simulink model "mpc_model_classical"  (R2019a)
settings: Solver=VariableStepAuto  StartTime=0.0  StopTime=Tfinal  RelTol=1e-3
values from neighbouring files (symbols this model uses):
  A = [-0.0285 -0.0014; -0.0371 -0.1476]    [model.m]
  DCLINK_Cap = 1000e-12    (= 1e-09)    [mpc_model_parameters.m]    (also in mpc_model_parameters_dual_module.m = 0.001)
  FaultTime = 50    [mpc_model_parameters.m]
  FluxPM = MeanInducedVoltagePeak/(2*pi*100)    [mpc_model_parameters.m]    (also in mpc_model_parameters_dual_module.m)
  Inertia = 1e-2    (= 0.01)    [mpc_model_parameters.m]    (also in mpc_model_parameters_dual_module.m)
  intangle1 = 0    [mpc_model_parameters.m]    (also in mpc_model_parameters_dual_module.m)
  Ki = 8    [mpc_model_parameters_dual_module.m]
  Kp = 0.8    [mpc_model_parameters_dual_module.m]
  ma = 0.9    [mpc_model_parameters.m]    (also in mpc_model_parameters_dual_module.m)
  MeanLd = (1/12)*(Module1Phase_A_Ld+Module1Phase_B_Ld+Module1Phase_C_Ld+     Module2Phase_A_Ld+Module2Phase_B_Ld+Module2Phase_C_Ld+     Module3Phase_A_Ld+Module3Phase_B_Ld+Module3Phase_C_Ld+     Module4Phase_A_Ld+Module4Phase_B_Ld+Module4Phase_C_Ld)    [mpc_model_parameters.m]    (also in mpc_model_parameters_dual_module.m)
  MeanLq = (1/12)*(Module1Phase_A_Lq+Module1Phase_B_Lq+Module1Phase_C_Lq+     Module2Phase_A_Lq+Module2Phase_B_Lq+Module2Phase_C_Lq+     Module3Phase_A_Lq+Module3Phase_B_Lq+Module3Phase_C_Lq+     Module4Phase_A_Lq+Module4Phase_B_Lq+Module4Phase_C_Lq)    [mpc_model_parameters.m]    (also in mpc_model_parameters_dual_module.m)
  PI_Frequency = 5000    [mpc_model_parameters_dual_module.m]
  PI_Sat = iqrated*2    [mpc_model_parameters_dual_module.m]
  PI_Ts = 1/PI_Frequency    (= 0.0002)    [mpc_model_parameters_dual_module.m]
  PolePairs = 10    [mpc_model_parameters.m]    (also in mpc_model_parameters_dual_module.m)
  ref_frequency = 100*pi    (= 314.159265359)    [mpc_model_parameters.m]    (also in mpc_model_parameters_dual_module.m)
  Rin = 1e-3    (= 0.001)    [mpc_model_parameters.m]    (also in mpc_model_parameters_dual_module.m)
  Rs = 0.531    [Loss_Distribution.m]    (also in MPC_id_iq.m; mpc_model_parameters.m = 0.321; mpc_model_parameters_dual_module.m = 0.539)
  Sampling_time = 1e-6    (= 1e-06)    [mpc_model_parameters.m]    (also in mpc_model_parameters_dual_module.m)
  SpeedRef1 = 50    [mpc_model_parameters.m]    (also in mpc_model_parameters_dual_module.m = 35)
  SpeedRef2 = 100    [mpc_model_parameters.m]    (also in mpc_model_parameters_dual_module.m = 35)
  SpeedRefUpdateTime = 0.25    [mpc_model_parameters.m]    (also in mpc_model_parameters_dual_module.m = 1.75)
  Tload1 = 5    [mpc_model_parameters.m]    (also in mpc_model_parameters_dual_module.m = 30)
  Tload2 = 10    [mpc_model_parameters.m]    (also in mpc_model_parameters_dual_module.m = 63.6619772368)
  TloadUpdateTime = 0.5    [mpc_model_parameters.m]    (also in mpc_model_parameters_dual_module.m)
  Vdc = 50    [mpc_model_parameters.m]    (also in mpc_model_parameters_dual_module.m = 40)
  Vin = Vdc + Rin*(Pout/Vdc)    (= 50.04)    [mpc_model_parameters.m]    (also in mpc_model_parameters_dual_module.m = 40.05)
  ViscousFriction = 1e-3    (= 0.001)    [mpc_model_parameters.m]    (also in mpc_model_parameters_dual_module.m)
undefined symbols (not defined in the file or in its folder): DiscIntNeverNeededParam
libraries: powerlib x16, dspswit3 x8, powerlib_meascontrol x5, simulink x1, dspsigops x1
settings Model: Creator=hakan  LastModifiedBy=hakan
settings SolverCC: ZeroCrossAlgorithm=Adaptive
settings DebuggingCC: IgnoredZcDiagnostic=none

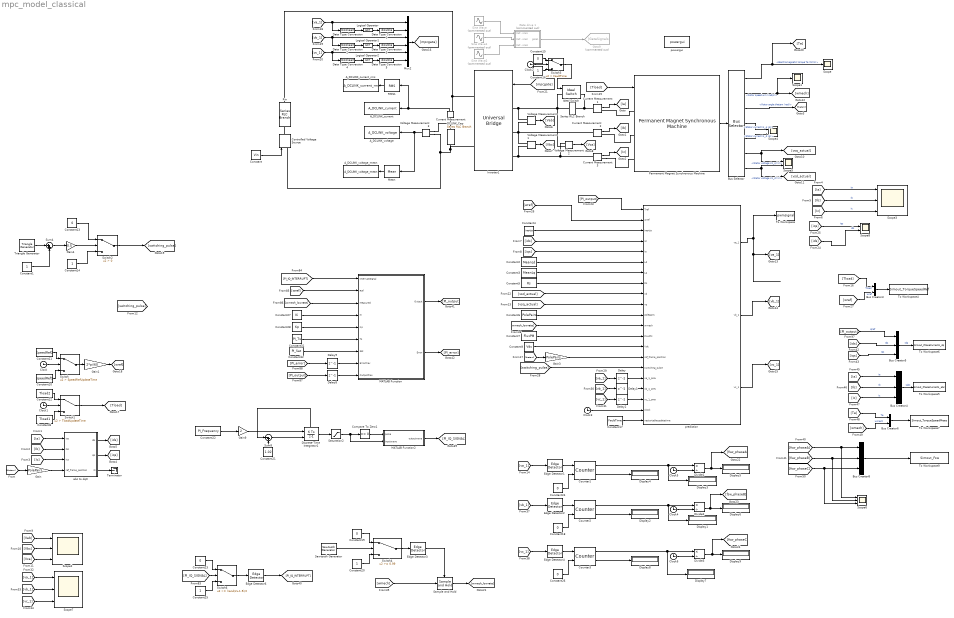
== system mpc_model_classical ==
  A_DCLINK_current : ToWorkspace  VariableName=A_DCLINK_current  SaveFormat=Structure With Time  SampleTime=-1
  A_DCLINK_current_rms : ToWorkspace  VariableName=A_DCLINK_current_rms  SaveFormat=Structure With Time  SampleTime=-1
  A_DCLINK_voltage : ToWorkspace  VariableName=A_DCLINK_voltage  SaveFormat=Structure With Time  SampleTime=-1
  A_DCLINK_voltage_mean : ToWorkspace  VariableName=A_DCLINK_voltage_mean  SaveFormat=Structure With Time  SampleTime=-1
  Bus Creator3 : BusCreator  Inputs=2
  Bus Creator4 : BusCreator  Inputs=3
  Bus Creator5 : BusCreator  Inputs=3
  Bus Creator6 : BusCreator  Inputs=2
  Bus Creator8 : BusCreator  Inputs=3
  Bus Selector : BusSelector  OutputSignals=Electromagnetic torque Te (N*m),Rotor speed wm (rad/s),Rotor angle thetam (rad),Stator current is_q (A),Stator current is_d (A),Stator voltage Vs_q (V),Stator voltage Vs_d (V)
  Clock{,1..6} (7 alike) : Clock
  Compare To Zero1 : simulink/Logic and Bit Operations/Compare To Zero  relop===  OutDataTypeStr=boolean
  Constant : Constant  Value=Vin
  Constant{1,14,16,20,25} (5 alike) : Constant
  Constant10 : Constant  Value=SpeedRef1
  Constant11 : Constant  Value=SpeedRef2
  Constant12 : Constant  Value=Tload2
  Constant{13,15,18..19,23..24,26} (7 alike) : Constant  Value=0
  Constant17 : Constant  Value=FaultTime
  Constant2 : Constant  Value=MeanLd
  Constant21 : Constant  Value=1.02
  Constant22 : Constant  Value=PI_Frequency
  Constant27 : Constant  Value=Ki
  Constant28 : Constant  Value=Kp
  Constant3 : Constant  Value=MeanLq
  Constant31 : Constant  Value=PI_Ts
  Constant32 : Constant  Value=PI_Sat
  Constant4 : Constant  Value=Inertia
  Constant5 : Constant  Value=Rs
  Constant6 : Constant  Value=PolePairs
  Constant7 : Constant  Value=FluxPM
  Constant8 : Constant  Value=Tload1
  Constant9 : Constant  Value=Vdc
  Controlled Voltage Source : powerlib/Electrical Sources/Controlled Voltage Source  Initialize=on  Source_Type=DC  Amplitude=0  Phase=0  Frequency=0  Measurements=None
      settings: SourceProductName=Simscape Electrical
  Counter1 : dspswit3/Counter  Direction=Up  CountEvent=Rising edge  CounterSize=User defined  MaxCount=9999999999999999999  InitialCount=0  Output=Count and Hit  HitValue=32  ResetInput=on  SamplesPerFrame=1  Ts=1  CntDtype=double  HitDtype=Logical
  Counter2 : dspswit3/Counter  Direction=Up  CountEvent=Rising edge  CounterSize=User defined  MaxCount=9999999999999999999  InitialCount=0  Output=Count and Hit  HitValue=32  ResetInput=on  SamplesPerFrame=1  Ts=1  CntDtype=double  HitDtype=Logical
  Counter3 : dspswit3/Counter  Direction=Up  CountEvent=Rising edge  CounterSize=User defined  MaxCount=9999999999999999999  InitialCount=0  Output=Count and Hit  HitValue=32  ResetInput=on  SamplesPerFrame=1  Ts=1  CntDtype=double  HitDtype=Logical
  Current Measurement{,1..3} (4 alike) : powerlib/Measurements/Current Measurement  PhasorSimulation=off  OutputType=Complex  PSBequivalent=0
      settings: SourceProductName=Simscape Electrical
  DCLINK_Cap : powerlib/Elements/Series RLC Branch  LConnTagsString=__new0  RConnTagsString=__new0  BranchType=C  Resistance=1  Inductance=1e-3  SetiL0=off  InitialCurrent=0  Capacitance=DCLINK_Cap  Setx0=on  InitialVoltage=Vin  Measurements=None
      settings: SourceProductName=Simscape Electrical
  Data Type Conversion : DataTypeConversion  OutDataTypeStr=boolean
  Data Type Conversion1 : DataTypeConversion  OutDataTypeStr=double
  Data Type Conversion2 : DataTypeConversion  OutDataTypeStr=boolean
  Data Type Conversion3 : DataTypeConversion  OutDataTypeStr=double
  Data Type Conversion4 : DataTypeConversion  OutDataTypeStr=boolean
  Data Type Conversion5 : DataTypeConversion  OutDataTypeStr=double
  Delay{,1..2,8..9} (5 alike) : Delay  DelayLength=1
  Discrete-Time Integrator1 : DiscreteIntegrator  ExternalReset=falling  SampleTime=Sampling_time  UpperSaturationLimit=1  LowerSaturationLimit=0  ShowStatePort=on  ICPrevOutput=DiscIntNeverNeededParam  ICPrevScaledInput=DiscIntNeverNeededParam
  Display{1..9} (9 alike) : Display
  Divide1 : Product  Inputs=*/
  Divide2 : Product  Inputs=*/
  Divide3 : Product  Inputs=*/
  Edge Detector{1..4,6} (5 alike) : dspswit3/Edge Detector  InputProcessing=Columns as channels (frame based)
      settings: SourceProductName=DSP System Toolbox  SourceProductBaseCode=DS
  Gain : Gain  Gain=PolePairs
  Gain1 : Gain  Gain=2*pi/60
  Gain3 : Gain  Gain=PolePairs
  Gain4 : Gain  Gain=0.5
  Gain9 : Gain  Gain=2
  Gate drive 1 : Subsystem  Commented=on
  Goto9 : Goto  Commented=on  GotoTag=GateSignals
  Ideal Switch : powerlib/Power Electronics/Ideal Switch  Ron=0.001  Lon=0  IC=0  Rs=1e5  Cs=inf  Measurements=on
      settings: SourceProductName=Simscape Electrical
  Inverter1 : powerlib/Power Electronics/Universal Bridge  Arms=3  SnubberResistance=1e5  SnubberCapacitance=inf  Device=IGBT / Diodes  Ron=0.65e-3  Lon=0  ForwardVoltages="[  0  0  ]"  ForwardVoltage=0  GTOparameters=[ 10e-6 , 20e-6 ]  IGBTparameters=[ 1e-6 , 2e-6 ]  Measurements=All voltages and currents  Measurements_2=None  converterType=Rectifier
      settings: SourceProductName=Simscape Electrical
  Logical Operator : Logic  Operator=NOT  AllPortsSameDT=off  OutDataTypeStr=boolean
  Logical Operator1 : Logic  Operator=NOT  AllPortsSameDT=off  OutDataTypeStr=boolean
  Logical Operator2 : Logic  Operator=NOT  AllPortsSameDT=off  OutDataTypeStr=boolean
  MATLAB Function : MATLAB Function  TreatAsAtomicUnit=on
  MATLAB Function2 : MATLAB Function  TreatAsAtomicUnit=on
  Mean : powerlib_meascontrol/Measurements/Mean  Freq=THD_mean_frequency  Vinit=0  Ts=0
      settings: SourceProductName=Simscape Electrical
  Mux2 : Mux  Inputs=6
  Permanent Magnet Synchronous Machine : powerlib/Machines/Permanent Magnet Synchronous Machine  NbPhases=3  FluxDistribution=Sinusoidal  RotorType=Round  MechanicalLoad=Torque Tm  PresetModel=No  ShowDetailedParameters=on  MeasurementBus=off  Resistance=Rs  Inductance=8.5e-3  dqInductances=[3.1e-3,3.6e-3]  La=Ls  MachineConstant=Voltage Constant (V_peak L-L / krpm)  Flux=0.18074  VoltageCst=VoltageConstant  TorqueCst=2.7111  Flat=120  Mechanical=[Inertia ViscousFriction PolePairs 0]  PolePairs=4  InitialConditions=[0,0, 0,0]  InitialConditions5ph=[0 0 0 0 0 0]  TsPowergui=0  TsBlock=-1  RefAngle=90 degrees behind phase A axis (modified Park)
  RMS1 : powerlib_meascontrol/Measurements/RMS  TrueRMS=on  Freq=Load_Nominal_Freq  RMSInit=10  Ts=0
      settings: SourceProductName=Simscape Electrical
  Rin : powerlib/Elements/Series RLC Branch  LConnTagsString=__new0  RConnTagsString=__new0  BranchType=R  Resistance=Rin  Inductance=1e-3  SetiL0=off  InitialCurrent=0  Capacitance=1000e-6  Setx0=off  InitialVoltage=0  Measurements=None
      settings: SourceProductName=Simscape Electrical
  Sample and Hold : dspsigops/Sample and Hold  trig=Rising edge  initCond=0  latchinput=off
  Saturation2 : Saturate  UpperLimit=1  LowerLimit=0
  Sawtooth Generator : powerlib_meascontrol/Pulse & Signal Generators/Sawtooth Generator  Freq=1000  Phase=180  Ts=0
      settings: SourceProductName=Simscape Electrical
  Scope : Scope
  Scope1 : Scope
  Scope{2..3,6..7} (4 alike) : Scope  NumInputPorts=3
  Scope4 : Scope  NumInputPorts=2
  Scope5 : Scope  NumInputPorts=2
  Scope8 : Scope  NumInputPorts=2
  Series RLC Branch : powerlib/Elements/Series RLC Branch  LConnTagsString=__new0  RConnTagsString=__new0  BranchType=R  Resistance=5000  Inductance=1e-3  SetiL0=off  InitialCurrent=0  Capacitance=1e-6  Setx0=off  InitialVoltage=0  Measurements=None
      settings: SourceProductName=Simscape Electrical
  Sine Wave : Sin  Commented=on  Amplitude=ma  Frequency=ref_frequency  SampleTime=0
  Sine Wave1 : Sin  Commented=on  Amplitude=ma  Frequency=ref_frequency  Phase=-2*pi/3  SampleTime=0
  Sine Wave2 : Sin  Commented=on  Amplitude=ma  Frequency=ref_frequency  Phase=2*pi/3  SampleTime=0
  Sum4 : Sum  Inputs=|++
  Sum8 : Sum  Inputs=|-+
  Switch : Switch  Criteria=u2 > Threshold  Threshold=SpeedRefUpdateTime
  Switch1 : Switch  Criteria=u2 > Threshold  Threshold=TloadUpdateTime
  Switch2 : Switch  Criteria=u2 > Threshold
  Switch3 : Switch  Criteria=u2 > Threshold  Threshold=FaultTime
  Switch4 : Switch  Threshold=0.99
  Switch6 : Switch  Threshold=(rand/2+1.5)/2
  Terminator : Terminator
  To Workspace : ToWorkspace  VariableName=pwmsignal  SaveFormat=Timeseries  SampleTime=-1
  To Workspace4 : ToWorkspace  VariableName=Simout_TorqueSpeedRef  SaveFormat=Timeseries  SampleTime=-1
  To Workspace5 : ToWorkspace  VariableName=Simout_PhaseCurrents_abc  SaveFormat=Timeseries  SampleTime=-1
  To Workspace6 : ToWorkspace  VariableName=Simout_PhaseCurrents_dq  SaveFormat=Timeseries  SampleTime=-1
  To Workspace7 : ToWorkspace  VariableName=Simout_TorqueSpeedMeas  SaveFormat=Timeseries  SampleTime=-1
  To Workspace9 : ToWorkspace  VariableName=Simout_Fsw  SaveFormat=Timeseries  SampleTime=-1
  Triangle Generator : powerlib_meascontrol/Pulse & Signal Generators/Triangle Generator  Freq=sw_frequency  Phase=0  Ts=Sampling_time
      settings: SourceProductName=Simscape Electrical
  Voltage Measurement{,1..3} (4 alike) : powerlib/Measurements/Voltage Measurement  PhasorSimulation=off  OutputType=Complex  PSBequivalent=0
      settings: SourceProductName=Simscape Electrical
  abc to dq0 : MATLAB Function  TreatAsAtomicUnit=on
  powergui : powerlib/powergui  Priority=1  SimulationMode=Discrete  SampleTime=Sampling_time  frequency=60  Iterations=50  frequencyindice=0  Pbase=100e6  ErrMax=1e-4  UnitsV=kV  UnitsW=MW  buscounter=0  FunctionMessages=off  echomessages=off  EnableUseOfTLC=off  CurrentSourceSwitches=off  DisableSnubberDevices=off  DisableRonSwitches=off  DisableVfSwitches=off  DisplayEquations=off  AutomaticDiscreteSolvers=off  SolverType=Tustin/Backward Euler (TBE)  Interpol=off  ExternalGateDelay=off  methode=off  Ts=100  x0status=blocks  SPID=on  SwTol=0  HookPort=off  NonlinearTolerance=0  nMaxIteration=15  ContinueOnMaxIteration=off  RestoreLinks=warning  ResistiveCurrentMeasurement=off  Frange=[0:2:500]  Ylog=off  Xlog=on  ShowGrid=off  save=off  variable=ZData  structure=0  ZoomFFT=off  StartTime=0.0  cycles=1  DisplayStyle=1  fundamental=60  FreqAxis=off  MaxFrequency=1000  frequencyindicesteady=1  RmsSteady=1  display=off
      settings: SourceProductName=Simscape Electrical
  prediction : MATLAB Function  TreatAsAtomicUnit=on
  wires:
  Voltage Measurement3/1 -> Mean/1, A_DCLINK_voltage/1
  RMS1/1 -> A_DCLINK_current_rms/1
  Constant/1 -> Controlled Voltage Source/1
  Mean/1 -> A_DCLINK_voltage_mean/1
  Current Measurement/1 -> RMS1/1, A_DCLINK_current/1
  Gate drive 1/1(gate1) -> Goto9/1
  Permanent Magnet Synchronous Machine/1 -> Bus Selector/1
  Bus Selector/1 -> [Te], Scope/1  "<Electromagnetic torque Te (N*m)>"
  Bus Selector/2 -> [wmech], Scope1/1  "<Rotor speed wm (rad/s)>"
  Sine Wave1/1 -> Gate drive 1/2(Reference2)
  Sine Wave/1 -> Gate drive 1/1(Reference1)
  Sine Wave2/1 -> Gate drive 1/3(Reference3)
  Current Measurement1/1 -> [Ia]
  Current Measurement2/1 -> [Ib]
  Current Measurement3/1 -> [Ic]
  Bus Selector/3 -> [thetam]  "<Rotor angle thetam (rad)>"
  [thetam] -> Gain/1
  [Ia] -> abc to dq0/1(ias)
  [Ib] -> abc to dq0/2(ibs)
  [Ic] -> abc to dq0/3(ics)
  Gain/1 -> abc to dq0/4(ref_frame_position)
  [Ia] -> Scope3/1  "Ia"
  [Ib] -> Scope3/2  "Ib"
  [Ic] -> Scope3/3  "Ic"
  Bus Selector/4 -> Scope4/1  "<Stator current is_q (A)>"
  Bus Selector/5 -> Scope4/2  "<Stator current is_d (A)>"
  abc to dq0/2(iqs) -> [iqs]
  abc to dq0/1(ids) -> [ids]
  abc to dq0/3(i0) -> Terminator/1
  [ids] -> prediction/4(id)
  [iqs] -> prediction/5(iq)
  Constant2/1 -> prediction/6(Ld)
  Constant3/1 -> prediction/7(Lq)
  Voltage Measurement/1 -> [Vab]
  Voltage Measurement1/1 -> [Vbc]
  Voltage Measurement2/1 -> [Vca]
  Bus Selector/6 -> Scope5/1, [vsq_actual]  "<Stator voltage Vs_q (V)>"
  Bus Selector/7 -> [vsd_actual], Scope5/2  "<Stator voltage Vs_d (V)>"
  [Vca] -> Scope2/3
  [Vbc] -> Scope2/2
  [Vab] -> Scope2/1
  [mpcgate] -> Inverter1/1
  Constant5/1 -> prediction/8(Rs)
  Constant6/1 -> prediction/11(polepairs)
  [wmech_lowrate] -> prediction/12(wmech)
  Constant7/1 -> prediction/13(FluxPM)
  prediction/2(vb_1) -> [vb_1]
  prediction/1(va_1) -> To Workspace/1, [va_1]
  prediction/3(vc_1) -> [vc_1]
  Constant9/1 -> prediction/14(Vdc)
  Gain3/1 -> prediction/15(ref_frame_position)
  [thetam] -> Gain3/1
  [va_1] -> Mux2/1, Data Type Conversion/1
  Logical Operator/1 -> Data Type Conversion1/1
  Data Type Conversion2/1 -> Logical Operator1/1
  Data Type Conversion3/1 -> Mux2/4
  Logical Operator2/1 -> Data Type Conversion5/1
  [vb_1] -> Mux2/3, Data Type Conversion2/1
  Logical Operator1/1 -> Data Type Conversion3/1
  [vc_1] -> Mux2/5, Data Type Conversion4/1
  Data Type Conversion5/1 -> Mux2/6
  Data Type Conversion1/1 -> Mux2/2
  Data Type Conversion4/1 -> Logical Operator2/1
  Data Type Conversion/1 -> Logical Operator/1
  Mux2/1 -> [mpcgate]
  [Tload] -> Permanent Magnet Synchronous Machine/1
  [vsq_actual] -> prediction/10(vq)
  [vsd_actual] -> prediction/9(vd)
  [iqs] -> Scope8/1  "iqs"
  [ids] -> Scope8/2  "ids"
  Constant4/1 -> prediction/3(Inertia)
  Constant10/1 -> Switch/3
  Constant11/1 -> Switch/1
  Switch/1 -> Gain1/1
  Clock/1 -> Switch/2
  Clock1/1 -> Switch1/2
  Constant12/1 -> Switch1/1
  Constant8/1 -> Switch1/3
  Switch1/1 -> [Tload]
  [wref] -> prediction/2(wref)
  Gain1/1 -> [wref]
  [Tload] -> Bus Creator3/1  "Tload"
  [wref] -> Bus Creator3/2  "wref"
  Bus Creator3/1 -> To Workspace4/1
  Sum4/1 -> Gain4/1
  Gain4/1 -> Switch2/2
  Triangle Generator/1 -> Sum4/1
  Constant1/1 -> Sum4/2
  Constant13/1 -> Switch2/1
  Constant14/1 -> Switch2/3
  Switch2/1 -> [switching_pulse]
  [switching_pulse] -> prediction/16(switching_pulse)
  Delay/1 -> prediction/17(va_1_prev)
  Delay1/1 -> prediction/18(vb_1_prev)
  Delay2/1 -> prediction/19(vc_1_prev)
  [va_1] -> Delay/1
  [vb_1] -> Delay1/1
  [vc_1] -> Delay2/1
  Clock2/1 -> Switch3/2
  Constant15/1 -> Switch3/1
  Constant16/1 -> Switch3/3
  Switch3/1 -> Ideal Switch/1
  Clock3/1 -> prediction/20(clock)
  Constant17/1 -> prediction/21(vectortableupdatetime)
  [va_1] -> Scope7/1
  [vb_1] -> Scope7/2
  [vc_1] -> Scope7/3
  Constant31/1 -> MATLAB Function/6(Ts)
  Delay8/1 -> MATLAB Function/9(OutputPrev)
  MATLAB Function/1(Output) -> [PI_output]
  [wref] -> MATLAB Function/2(Ref)
  Constant28/1 -> MATLAB Function/5(Kp)
  Delay9/1 -> MATLAB Function/8(ErrorPrev)
  Constant32/1 -> MATLAB Function/7(Sat)
  [PI_IQ_INTERRUPT] -> MATLAB Function/1(InterruptSignal)
  [wmech_lowrate] -> MATLAB Function/3(Measured)
  [PI_output] -> Delay8/1
  MATLAB Function/2(Error) -> [PI_error]
  Constant27/1 -> MATLAB Function/4(Ki)
  [PI_error] -> Delay9/1
  Constant22/1 -> Gain9/1
  MATLAB Function2/1(outputwave) -> [PI_IQ_SIGNAL]
  Discrete-Time Integrator1/1 -> Saturation2/1
  Saturation2/1 -> Compare To Zero1/1, MATLAB Function2/2(inputwave)
  Discrete-Time Integrator1/State -> Sum8/1
  Sum8/1 -> Discrete-Time Integrator1/2
  Compare To Zero1/1 -> MATLAB Function2/1(pulse)
  Gain9/1 -> Discrete-Time Integrator1/1
  Constant21/1 -> Sum8/2
  [PI_output] -> prediction/1(Tref)
  Constant20/1 -> Switch4/3
  Switch4/1 -> Edge Detector3/1
  Sawtooth Generator/1 -> Switch4/2
  Sample and Hold/1 -> [wmech_lowrate]
  [wmech] -> Sample and Hold/1
  Edge Detector3/1 -> Sample and Hold/Trigger
  Constant19/1 -> Switch4/1
  Switch6/1 -> Edge Detector6/1
  Edge Detector6/1 -> [PI_IQ_INTERRUPT]
  Constant23/1 -> Switch6/1
  Constant25/1 -> Switch6/3
  [PI_IQ_SIGNAL] -> Switch6/2
  Divide1/1 -> [fsw_phaseA], Display5/1
  Clock5/1 -> Divide1/2
  Counter1/2 -> Display4/1
  Counter1/1 -> Display3/1, Divide1/1
  Constant24/1 -> Counter1/2
  Edge Detector1/1 -> Counter1/1
  Constant18/1 -> Counter2/2
  Counter2/2 -> Display2/1
  Edge Detector2/1 -> Counter2/1
  Clock4/1 -> Divide2/2
  Counter2/1 -> Display1/1, Divide2/1
  Divide2/1 -> [fsw_phaseB], Display6/1
  Counter3/1 -> Divide3/1, Display7/1
  Edge Detector4/1 -> Counter3/1
  Clock6/1 -> Divide3/2
  Counter3/2 -> Display8/1
  Constant26/1 -> Counter3/2
  Divide3/1 -> [fsw_phaseC], Display9/1
  [va_1] -> Edge Detector1/1
  [vb_1] -> Edge Detector2/1
  [vc_1] -> Edge Detector4/1
  Bus Creator4/1 -> To Workspace5/1  "Iabc"
  [Ib] -> Bus Creator4/2  "Ib"
  [iqs] -> Bus Creator5/3  "iqs"
  [ids] -> Bus Creator5/2  "ids"
  [Ic] -> Bus Creator4/3  "Ic"
  [wmech] -> Bus Creator6/2  "wmech"
  [Te] -> Bus Creator6/1  "Te"
  [Ia] -> Bus Creator4/1  "Ia"
  Bus Creator8/1 -> To Workspace9/1
  [PI_output] -> Bus Creator5/1  "iqref"
  Bus Creator6/1 -> To Workspace7/1
  Bus Creator5/1 -> To Workspace6/1  "Idq"
  [fsw_phaseA] -> Scope6/1, Bus Creator8/1
  [fsw_phaseB] -> Scope6/2, Bus Creator8/2
  [fsw_phaseC] -> Scope6/3, Bus Creator8/3
  connections:
  Rin/LConn1 -- Current Measurement/RConn1 -- Inverter1/RConn1
  Controlled Voltage Source/LConn1 -- DCLINK_Cap/RConn1 -- Inverter1/RConn2 -- Voltage Measurement3/LConn2
  DCLINK_Cap/LConn1 -- Current Measurement/LConn1 -- Voltage Measurement3/LConn1
  Controlled Voltage Source/RConn1 -- Rin/RConn1
  Voltage Measurement2/LConn2 -- Ideal Switch/LConn1 -- Series RLC Branch/LConn1 -- Voltage Measurement/LConn1 -- Inverter1/LConn1
  Current Measurement2/LConn1 -- Voltage Measurement1/LConn1 -- Voltage Measurement/LConn2 -- Inverter1/LConn2
  Inverter1/LConn3 -- Voltage Measurement1/LConn2 -- Voltage Measurement2/LConn1 -- Current Measurement3/LConn1
  Current Measurement3/RConn1 -- Permanent Magnet Synchronous Machine/LConn3
  Permanent Magnet Synchronous Machine/LConn2 -- Current Measurement2/RConn1
  Permanent Magnet Synchronous Machine/LConn1 -- Current Measurement1/RConn1
  Current Measurement1/LConn1 -- Ideal Switch/RConn1 -- Series RLC Branch/RConn1

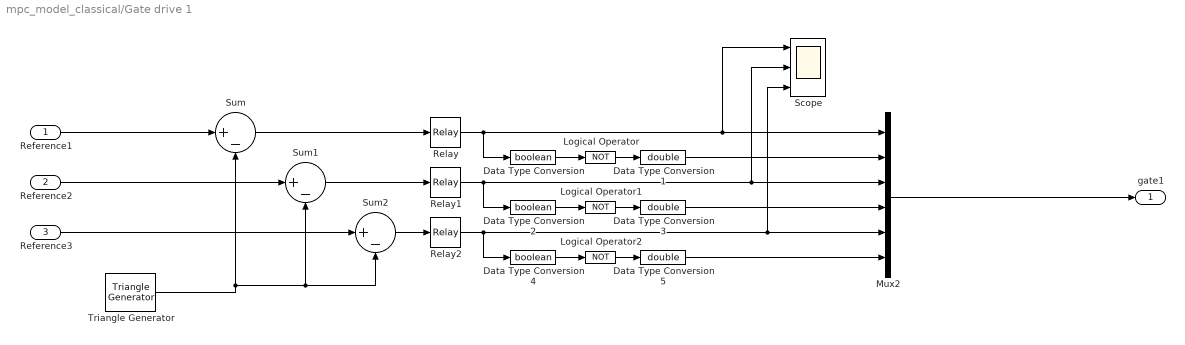
== system mpc_model_classical/Gate drive 1 ==
  Reference1 : Inport
  Reference2 : Inport  Port=2
  Reference3 : Inport  Port=3
  Data Type Conversion : DataTypeConversion  OutDataTypeStr=boolean
  Data Type Conversion1 : DataTypeConversion  OutDataTypeStr=double
  Data Type Conversion2 : DataTypeConversion  OutDataTypeStr=boolean
  Data Type Conversion3 : DataTypeConversion  OutDataTypeStr=double
  Data Type Conversion4 : DataTypeConversion  OutDataTypeStr=boolean
  Data Type Conversion5 : DataTypeConversion  OutDataTypeStr=double
  Logical Operator : Logic  Operator=NOT  AllPortsSameDT=off  OutDataTypeStr=boolean
  Logical Operator1 : Logic  Operator=NOT  AllPortsSameDT=off  OutDataTypeStr=boolean
  Logical Operator2 : Logic  Operator=NOT  AllPortsSameDT=off  OutDataTypeStr=boolean
  Mux2 : Mux  Inputs=6
  Relay : Relay
  Relay1 : Relay
  Relay2 : Relay
  Scope : Scope  NumInputPorts=3
  Sum : Sum  Inputs=|+-
  Sum1 : Sum  Inputs=|+-
  Sum2 : Sum  Inputs=|+-
  Triangle Generator : powerlib_meascontrol/Pulse & Signal Generators/Triangle Generator  Freq=sw_frequency  Phase=intangle1  Ts=Sampling_time
      settings: SourceProductName=Simscape Electrical
  gate1 : Outport
  wires:
  Mux2/1 -> gate1/1
  Data Type Conversion5/1 -> Mux2/6
  Logical Operator2/1 -> Data Type Conversion5/1
  Relay2/1 -> Scope/3, Mux2/5, Data Type Conversion4/1
  Data Type Conversion4/1 -> Logical Operator2/1
  Data Type Conversion3/1 -> Mux2/4
  Logical Operator1/1 -> Data Type Conversion3/1
  Relay1/1 -> Scope/2, Mux2/3, Data Type Conversion2/1
  Data Type Conversion2/1 -> Logical Operator1/1
  Data Type Conversion1/1 -> Mux2/2
  Logical Operator/1 -> Data Type Conversion1/1
  Relay/1 -> Scope/1, Mux2/1, Data Type Conversion/1
  Data Type Conversion/1 -> Logical Operator/1
  Sum2/1 -> Relay2/1
  Sum1/1 -> Relay1/1
  Sum/1 -> Relay/1
  Reference3/1 -> Sum2/1
  Reference2/1 -> Sum1/1
  Triangle Generator/1 -> Sum/2, Sum2/2, Sum1/2
  Reference1/1 -> Sum/1

== matlab function mpc_model_classical/prediction ==
  data: Tref input; wref input; Inertia input; id input; iq input; Ld input; Lq input; Rs input; vd input; vq input; polepairs input; wmech input; FluxPM input; va_1 output; vb_1 output; vc_1 output; Vdc input; ref_frame_position input; switching_pulse input; va_1_prev input; vb_1_prev input; vc_1_prev input; clock input; vectortableupdatetime input
function [va_1, vb_1,vc_1 ]  = fcn(Tref,wref,Inertia,id, iq, Ld, Lq, Rs,vd, vq,polepairs,wmech,FluxPM,Vdc,ref_frame_position,switching_pulse,va_1_prev, vb_1_prev,vc_1_prev,clock,vectortableupdatetime)
VoltageVector = [0 0 0; 0 0 1; 0 1 0; 0 1 1; 1 0 0; 1 0 1; 1 1 0; 1 1 1];
Ts = 1e-6;
% Ts = 1/40000;
% id_1 = id + Ts*(vd/Ld-Rs/Ld*id+Lq/Ld*polepairs*wmech*iq);
% iq_1 = iq + Ts*(vq*Lq-Rs/Lq*iq-Ld/Lq*polepairs*wmech*id-FluxPM*polepairs*wmech/Lq);
% Te_1 = 1.5*polepairs*(FluxPM*iq_1+0*(Ld-Lq)*id_1*iq_1);
% iqs = (vqs-fluxlinkage_qs_derivative-ref_frame_velocity*fluxlinkage_ds)/rs;
% ids = (vds-fluxlinkage_ds_derivative+ref_frame_velocity*fluxlinkage_qs)/rs;

cost = zeros(1,8);
vectortobeapplied = zeros(1,3);
wref = 200*2*pi/60;
for i = 1:8
    %get the vectors
    if(clock>vectortableupdatetime)
        va = 1;
        vb = VoltageVector(i,2);
        vc = VoltageVector(i,3);        
    else
        va = VoltageVector(i,1);
        vb = VoltageVector(i,2);
        vc = VoltageVector(i,3);        
    end
        

    %calculate  vd vq v0
    vds = Vdc*2/3*(va*sin(ref_frame_position)+vb*sin(ref_frame_position-2*pi/3)+vc*sin(ref_frame_position+2*pi/3));
    vqs =  Vdc*2/3*(va*cos(ref_frame_position)+vb*cos(ref_frame_position-2*pi/3)+vc*cos(ref_frame_position+2*pi/3));
    v0 = Vdc*2/3*1/2*(va+vb+vc);
    %predict the future output
    id_1 = id + Ts*(vds/Ld-Rs/Ld*id+Lq/Ld*polepairs*wmech*iq);
    iq_1 = iq + Ts*(vqs*Lq-Rs/Lq*iq-Ld/Lq*polepairs*wmech*id-FluxPM*polepairs*wmech/Lq);
    Te_1 = 1.5*polepairs*(FluxPM*iq_1+0*(Ld-Lq)*id_1*iq_1); % reluctance torque component is multiplied by 0, since it caused unreasonable torque values.
    
    id_2 = id_1 + Ts*(vds/Ld-Rs/Ld*id_1+Lq/Ld*polepairs*wmech*iq_1);
    iq_2 = iq_1 + Ts*(vqs*Lq-Rs/Lq*iq_1-Ld/Lq*polepairs*wmech*id_1-FluxPM*polepairs*wmech/Lq);    
    
    wmech_1 = wmech + Ts*(Te_1-Tref)*Inertia;
    %calculate the cost
%     if(abs(iq)>30)||(abs(Te_1)>50)
% %         protection = inf;
%     else
        protection = 0;
%     end
    cost(i) = 3000000000*abs(Tref-iq_2)^2+abs(id_2)^2*150000+protection;
%     cost(i) = 100000000*abs(wref-wmech_1)+abs(id_1)*1500+protection;

end

[mincostval, index] = min(cost);
% apply the one with minimum cost
vectortobeapplied(1) = VoltageVector(index,1);
vectortobeapplied(2) = VoltageVector(index,2);
vectortobeapplied(3) = VoltageVector(index,3);


if(switching_pulse==1)
    va_1 = vectortobeapplied(1);
    vb_1 = vectortobeapplied(2);
    vc_1 = vectortobeapplied(3);
else
    va_1 = va_1_prev;
    vb_1 = vb_1_prev;
    vc_1 = vc_1_prev;    
end

== matlab function mpc_model_classical/MATLAB Function2 ==
  data: pulse input; inputwave input; outputwave output
function outputwave  = fcn(pulse, inputwave)

persistent state

if isempty(state)
state = 0;
end

if(pulse==1)
    state = state +1;
end

if(mod(state,2)==1)
    outputwave = inputwave;
    return;
end
if(mod(state,2)==0)
    outputwave = 1-inputwave;
    return;
end

outputwave = 5;

== matlab function mpc_model_classical/MATLAB Function ==
  data: InterruptSignal input; Ref input; Measured input; Ki input; Output output; Kp input; Ts input; Sat input; Error output; ErrorPrev input; OutputPrev input
function [Output,Error] = fcn(InterruptSignal,Ref,Measured,Ki,Kp,Ts,Sat, ErrorPrev,OutputPrev)
Error=0;
Output = 0;

if(InterruptSignal ==1)
    Error = Ref-Measured;
    
    Output = OutputPrev + Kp*(Error-ErrorPrev)+Ts/2*Ki*((Error+ErrorPrev));
    %  iqref = iqref_prev + Kp*(Speed_Error-Speed_Error_prev)+Ts_PI/2*Ki*((Speed_Error+Speed_Error_prev));
    if(abs(Output)>(Sat))
        if(Output>0)
            Output = Sat;
        else
            Output = -(Sat);
        end
    end
else
    Output=OutputPrev;
    Error = ErrorPrev;
end

== matlab function mpc_model_classical/abc to dq0 ==
  data: ids output; iqs output; ias input; ibs input; ics input; ref_frame_position input; i0 output
function [ids,iqs,i0 ]  = fcn(ias,ibs,ics,ref_frame_position)





ids = 2/3*(ias*sin(ref_frame_position)+ibs*sin(ref_frame_position-2*pi/3)+ics*sin(ref_frame_position+2*pi/3));
iqs =  2/3*(ias*cos(ref_frame_position)+ibs*cos(ref_frame_position-2*pi/3)+ics*cos(ref_frame_position+2*pi/3));
i0 = 2/3*1/2*(ias+ibs+ics);
% iqs = (vqs-fluxlinkage_qs_derivative-ref_frame_velocity*fluxlinkage_ds)/rs;
% ids = (vds-fluxlinkage_ds_derivative+ref_frame_velocity*fluxlinkage_qs)/rs;
